simulink model "effektforstarker"  (Simulink 7.4)
settings: Solver=ode4  StartTime=0.0  StopTime=inf  FixedStep=0.1  RelTol=1e-3
libraries: xpcnilib x2, xpclib x2, simulink x1
settings Model: Creator=Skov  LastModifiedBy=Skov  SimulationMode=external  BufferReuse=off
settings DataIOCC: SaveState=on  InspectSignalLogs=on
settings OptimizationCC: BlockReduction=off  OptimizeBlockIOStorage=off  BufferReuse=off  ExpressionFolding=off  LocalBlockOutputs=off
settings HardwareCC: ProdIntDivRoundTo=Zero  ProdEndianess=LittleEndian  ProdHWDeviceType=Generic->32-bit x86 compatible
settings RTWCC: SystemTargetFile=xpctarget.tlc  TemplateMakefile=xpc_default_tmf  Description=xPC Target  ProcessScript=xpctarget_make_rtw_hook  RTWCompilerOptimization=On
settings xpcTargetCC: TargetFcnLib=ansi_tfl_table_tmw.mat  TargetFunctionLibrary=ANSI_C  ParMdlRefBuildCompliant=off  PortableWordSizes=off  xPCLoadParamSetFile=off

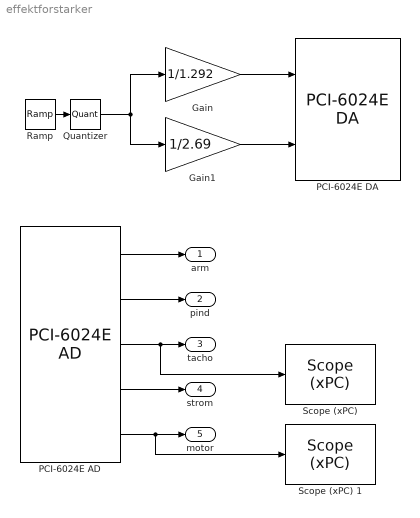
== system effektforstarker ==
  Gain : Gain  Gain=1/1.292  ParameterDataType=fixdt(1, 16)  ParameterScaling=2^0  OutDataType=fixdt(1, 16)  OutScaling=2^0
  Gain1 : Gain  Gain=1/2.69  ParameterDataType=fixdt(1, 16)  ParameterScaling=2^0  OutDataType=fixdt(1, 16)  OutScaling=2^0
  PCI-6024E AD : xpcnilib/A//D/E Series/PCI-6024E AD  channel=[1 2 3 4 5]  range=[-10]  coupling=[0]  sampletime=0.1  slot=-1
  PCI-6024E DA : xpcnilib/D//A/E Series/PCI-6024E DA  channel=[1 2]  reset=[1]  initValue=[0]  sampletime=0.1  slot=-1
  Quantizer : Quantizer  QuantizationInterval=0.1  LinearizeAsGain=off
  Ramp : simulink/Sources/Ramp  SystemSampleTime=-1  slope=0.02  start=2.5  X0=-5
  "Scope (xPC) " : xpclib/Misc./Scope (xPC)   SystemSampleTime=-1  scopeno=1  scopetype=Target  autostart=on  viewmode=Numerical  formatstr='%15.6f'  grid=on  ylimits=[-5,5]  nosamples=250  noprepostsamples=0  interleave=1  triggermode=FreeRun  triggersignal=1  triggerlevel=0.0  triggerslope=Either  triggerscope=1  triggersample=0  filename=data.dat  mode=Lazy  writesize=512  autorestart=off  dynamicfilemode=off  maxwritefilesize=512*1024^2
  Scope (xPC) 1 : xpclib/Misc./Scope (xPC)   SystemSampleTime=-1  scopeno=2  scopetype=Target  autostart=on  viewmode=Numerical  formatstr='%15.6f'  grid=on  ylimits=[-5,5]  nosamples=250  noprepostsamples=0  interleave=1  triggermode=FreeRun  triggersignal=1  triggerlevel=0.0  triggerslope=Either  triggerscope=1  triggersample=0  filename=data.dat  mode=Lazy  writesize=512  autorestart=off  dynamicfilemode=off  maxwritefilesize=512*1024^2
  arm : Outport  OutDataType=fixdt(1, 16)  OutScaling=2^0
  pind : Outport  Port=2  OutDataType=fixdt(1, 16)  OutScaling=2^0
  tacho : Outport  Port=3  OutDataType=fixdt(1, 16)  OutScaling=2^0
  strom : Outport  Port=4  OutDataType=fixdt(1, 16)  OutScaling=2^0
  motor : Outport  Port=5  OutDataType=fixdt(1, 16)  OutScaling=2^0
  wires:
  PCI-6024E AD/1 -> arm/1
  PCI-6024E AD/2 -> pind/1
  PCI-6024E AD/3 -> tacho/1, "Scope (xPC) "/1
  Gain1/1 -> PCI-6024E DA/2
  Gain/1 -> PCI-6024E DA/1
  Ramp/1 -> Quantizer/1
  PCI-6024E AD/4 -> strom/1
  PCI-6024E AD/5 -> motor/1, Scope (xPC) 1/1
  Quantizer/1 -> Gain/1, Gain1/1
